simulink model "adjoint_of_homingLoopPNG_2"  (Simulink 7.1)
settings: Solver=ode45  StartTime=0.0  StopTime=TFINAL-0.0001  MaxStep=0.01  RelTol=1e-3
values from neighbouring files (symbols this model uses):
  AT = 3    [linearizedPNG_ini.m]    (also in missdisatnce_adjoint.m; missdistance_homing_loop.m; missdistance_linearized.m; truePNG_ini.m = 0)
  HE = 0*(-30/180*pi)    (= 0)    [linearizedPNG_ini.m]    (also in missdisatnce_adjoint.m = 0.523598775598; missdistance_homing_loop.m; missdistance_linearized.m)
  Tautopilot = 0    [linearizedPNG_ini.m]    (also in missdisatnce_adjoint.m = 2; missdistance_homing_loop.m = 2; missdistance_linearized.m = 2; truePNG_ini.m = 0.2)
  VC = VM+VT    (= 140)    [linearizedPNG_ini.m]
  VM = 100    [linearizedPNG_ini.m]    (also in truePNG_ini.m = 0.5)
settings Model: Creator=LESSONS  LastModifiedBy=LESSONS
settings DebuggingCC: SolverPrmCheckMsg=none

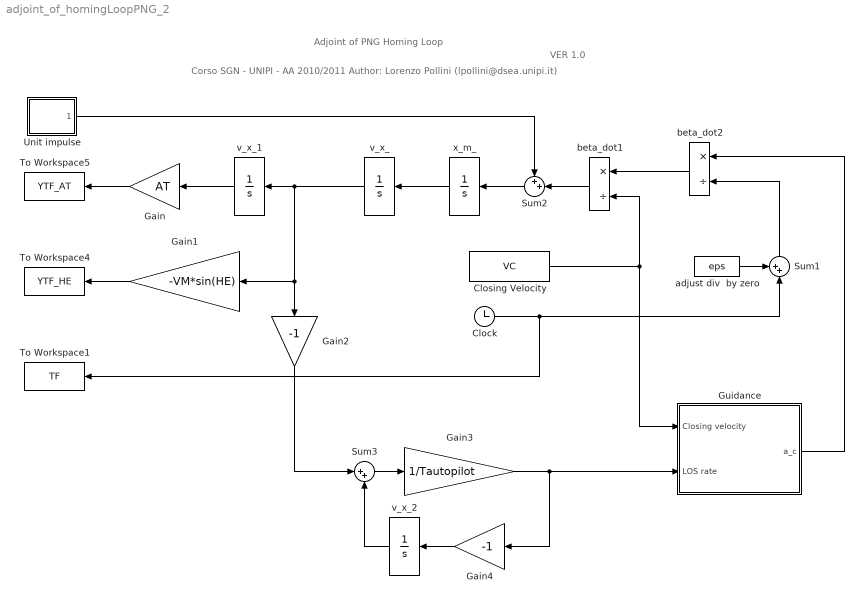
== system adjoint_of_homingLoopPNG_2 ==
  note: Adjoint of PNG Homing Loop
  note: Corso SGN - UNIPI - AA 2010/2011
      | Author: Lorenzo Pollini (lpollini@dsea.unipi.it)
  note: VER 1.0
  Clock : Clock
      settings: Decimation=10
  Closing Velocity : Constant  Value=VC  OutDataType=sfix(16)  OutScaling=2^0
  Gain : Gain  Orientation=left  Gain=AT  ParameterDataType=sfix(16)  ParameterScaling=2^0  OutDataType=sfix(16)  OutScaling=2^0
  Gain1 : Gain  Orientation=left  Gain=-VM*sin(HE)  ParameterDataType=sfix(16)  ParameterScaling=2^0  OutDataType=sfix(16)  OutScaling=2^0
  Gain2 : Gain  Orientation=down  Gain=-1  ParameterDataType=sfix(16)  ParameterScaling=2^0  OutDataType=sfix(16)  OutScaling=2^0
  Gain3 : Gain  Gain=1/Tautopilot  ParameterDataType=sfix(16)  ParameterScaling=2^0  OutDataType=sfix(16)  OutScaling=2^0
  Gain4 : Gain  Orientation=left  Gain=-1  ParameterDataType=sfix(16)  ParameterScaling=2^0  OutDataType=sfix(16)  OutScaling=2^0
  Guidance : Subsystem
  Sum1 : Sum  Orientation=up  Inputs=++|  OutDataType=sfix(16)  OutScaling=2^0
  Sum2 : Sum  Orientation=left  Inputs=++|  OutDataType=sfix(16)  OutScaling=2^0
  Sum3 : Sum  Inputs=|++  OutDataType=sfix(16)  OutScaling=2^0
  To Workspace1 : ToWorkspace  VariableName=TF  SampleTime=-1  SaveFormat=Structure With Time
  To Workspace4 : ToWorkspace  VariableName=YTF_HE  SampleTime=-1  SaveFormat=Structure With Time
  To Workspace5 : ToWorkspace  VariableName=YTF_AT  SampleTime=-1  SaveFormat=Structure With Time
  Unit impulse : Subsystem
  adjust div  by zero : Constant  Value=eps  OutDataType=sfix(16)  OutScaling=2^0
  beta_dot1 : Product  Orientation=left  Inputs=*/  OutDataType=sfix(16)  OutScaling=2^-10
  beta_dot2 : Product  Orientation=left  Inputs=*/  OutDataType=sfix(16)  OutScaling=2^-10
  v_x_ : Integrator  Orientation=left
  v_x_1 : Integrator  Orientation=left
  v_x_2 : Integrator  Orientation=left
  x_m_ : Integrator  Orientation=left
  wires:
  Closing Velocity/1 -> Guidance/1(Closing velocity), beta_dot1/2
  Clock/1 -> To Workspace1/1, Sum1/2
  v_x_/1 -> Gain1/1, Gain2/1, v_x_1/1
  v_x_1/1 -> Gain/1
  x_m_/1 -> v_x_/1
  beta_dot2/1 -> beta_dot1/1
  Sum2/1 -> x_m_/1
  beta_dot1/1 -> Sum2/2
  Unit impulse/1(impulse) -> Sum2/1
  Gain/1 -> To Workspace5/1
  Gain1/1 -> To Workspace4/1
  Gain2/1 -> Sum3/1
  Guidance/1(a_c) -> beta_dot2/1
  Sum1/1 -> beta_dot2/2
  adjust div  by zero/1 -> Sum1/1
  Sum3/1 -> Gain3/1
  v_x_2/1 -> Sum3/2
  Gain4/1 -> v_x_2/1
  Gain3/1 -> Gain4/1, Guidance/2(LOS rate)

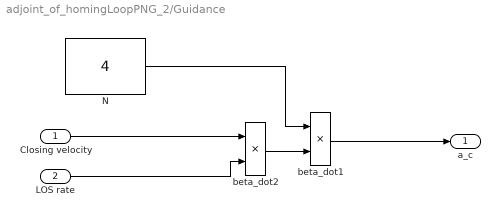
== system adjoint_of_homingLoopPNG_2/Guidance ==
  Closing velocity : Inport  OutDataType=sfix(16)  OutScaling=2^0
  LOS rate : Inport  Port=2  OutDataType=sfix(16)  OutScaling=2^0
  N : Constant  Value=4  OutDataType=sfix(16)  OutScaling=2^0
  beta_dot1 : Product  Inputs=**  OutDataType=sfix(16)  OutScaling=2^-10
  beta_dot2 : Product  Inputs=**  OutDataType=sfix(16)  OutScaling=2^-10
  a_c : Outport  OutDataType=sfix(16)  OutScaling=2^0
  wires:
  Closing velocity/1 -> beta_dot2/1
  beta_dot1/1 -> a_c/1
  LOS rate/1 -> beta_dot2/2
  beta_dot2/1 -> beta_dot1/2
  N/1 -> beta_dot1/1

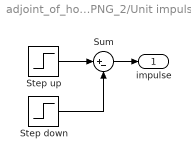
== system adjoint_of_homingLoopPNG_2/Unit impulse ==
  Step down : Step  Time=eps  After=1/eps  SampleTime=0
  Step up : Step  Time=0  After=1/eps  SampleTime=0
  Sum : Sum  Inputs=|+-  OutDataType=sfix(16)  OutScaling=2^0
  impulse : Outport
  wires:
  Step up/1 -> Sum/1
  Step down/1 -> Sum/2
  Sum/1 -> impulse/1
